simulink model "pitchShifter"  (R2020a)
settings: Solver=FixedStepAuto  StartTime=0.0  StopTime=386.015  FixedStep=1/4000  RelTol=1e-3  EnableMultiTasking=on
settings Model: Creator=Ivan Vican  LastModifiedBy=Korisnik
settings DataIOCC: LimitDataPoints=on  SaveFormat=Array  ReturnWorkspaceOutputs=off
settings OptimizationCC: ZeroExternalMemoryAtStartup=off  ZeroInternalMemoryAtStartup=off  LifeSpan=inf
settings DebuggingCC: SFUnexpectedBacktrackingDiag=warning  SFNoUnconditionalDefaultTransitionDiag=warning  ArithmeticOperatorsInVariantConditions=warning
settings HardwareCC: ProdBitPerPointer=32  ProdBitPerSizeT=32  ProdBitPerPtrDiffT=32  ProdLargestAtomicFloat=None  ProdIntDivRoundTo=Undefined  ProdEndianess=Unspecified  ProdWordSize=32  ProdHWDeviceType=32-bit Generic
settings ModelReferenceCC: PropagateSignalLabelsOutOfModel=off
settings SFSimCC: SimUseLocalCustomCode=off  CustomCodeUndefinedFunction=UseInterfaceOnly
settings RTWCC: RTWUseLocalCustomCode=off  TargetLang=C++
settings CodeAppCC: StateflowObjectComments=on
settings GRTTargetCC: TargetLangStandard=C89/C90 (ANSI)  MatFileLogging=off  MultiInstanceERTCode=on  CodeInterfacePackaging=C++ class
settings ConfigComp: CovMetricSettings=dw  CovHtmlReporting=on  CovSaveCumulativeToWorkspaceVar=on  CovSaveSingleToWorkspaceVar=on  CovExternalEMLEnable=off

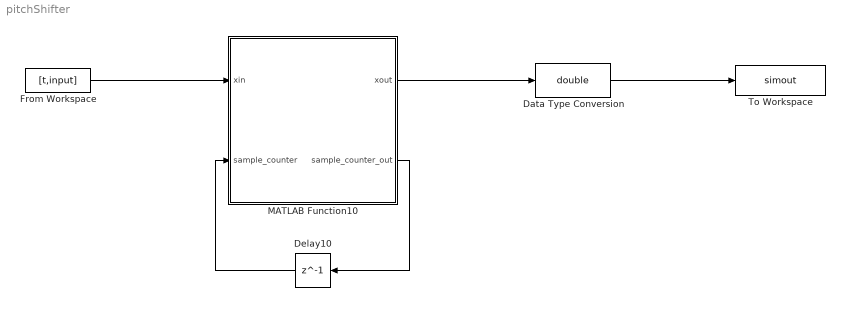
== system pitchShifter ==
  Data Type Conversion : DataTypeConversion  OutDataTypeStr=double
  Delay10 : Delay  DelayLength=1  InitialCondition=1
  From Workspace : FromWorkspace  VariableName=[t,input]  SampleTime=1/4000
  MATLAB Function10 : MATLAB Function  TreatAsAtomicUnit=on
  To Workspace : ToWorkspace  VariableName=simout  SampleTime=-1
      settings: Save2DSignal=2-D array (concatenate along first dimension)
  wires:
  Delay10/1 -> MATLAB Function10/2(sample_counter)
  MATLAB Function10/2(sample_counter_out) -> Delay10/1
  Data Type Conversion/1 -> To Workspace/1
  MATLAB Function10/1(xout) -> Data Type Conversion/1
  From Workspace/1 -> MATLAB Function10/1(xin)

== matlab function pitchShifter/MATLAB Function10 ==
  data: xin input; xout output; sample_counter input; sample_counter_out output
function [xout,sample_counter_out] = pitch24(xin,sample_counter)

persistent frame;
persistent frame_buff;
persistent frame_cnt;
persistent outputVector;
persistent pitchPrev;
persistent phaseCumulative;
persistent previousPhase;
persistent all;

% Window size
winSize = 128*2;
% Space between windows
hop = 8*2;
% Pitch scaling factor
alpha = 2^(24/12);
% Intermediate constants
hopOut = round(alpha*hop);

if isempty(frame)    
     frame = zeros([1,hop]);
     frame_buff = zeros([1,winSize]);
     frame_cnt = 0;
     outputVector = zeros([1,winSize]);
     pitchPrev = zeros([winSize/hop,winSize]);
     phaseCumulative = zeros(1,winSize);
     previousPhase = zeros(1,winSize);
     all = zeros([1,hop]);
end

frame(sample_counter) = xin;
xout = all(sample_counter);

% Intermediate constants
hopOut = round(alpha*hop);

% Hanning window for overlap-add
wn = hann(winSize*2+1);
wn = wn(2:2:end);

if sample_counter == hop
%% Initialization

% Create a frame matrix for the current input

% for i=1:winSize/hop-1
% pitchPrev(i,:) = pitchPrev(i+1,:);
% end

frame_cnt = frame_cnt + 1;

frame_buff = [frame_buff(hop+1:winSize) frame];
currentFrame = frame_buff;
    
%% Analysis
    
    % Window the frame
    currentFrameWindowed = currentFrame .* wn' / sqrt(((winSize/hop)/2));
    
    % Get the FFT
    currentFrameWindowedFFT = fft(currentFrameWindowed);
    
    % Get the magnitude
    magFrame = abs(currentFrameWindowedFFT);
    
    % Get the angle
    phaseFrame = angle(currentFrameWindowedFFT);
    
%% Processing    

    % Get the phase difference
    deltaPhi = phaseFrame - previousPhase;
    previousPhase = phaseFrame;
    
    % Remove the expected phase difference
    deltaPhiPrime = deltaPhi - hop * 2*pi*(0:(winSize-1))/winSize;
    
    % Map to -pi/pi range
    deltaPhiPrimeMod = mod(deltaPhiPrime+pi, 2*pi) - pi;
     
    % Get the true frequency
    trueFreq = 2*pi*(0:(winSize-1))/winSize + deltaPhiPrimeMod/hop;

    % Get the final phase
    phaseCumulative = phaseCumulative + hopOut * trueFreq;    
   
%% Synthesis    
    
    % Get the magnitude
    outputMag = magFrame;
    
    % Produce output frame
    outputFrame = real(ifft(outputMag .* exp(j*phaseCumulative)));
     
    % Save frame that has been processed
    outputy = outputFrame .* wn' / sqrt(((winSize/hopOut)/2));
       
  outputVector = outputy;
end

if (sample_counter == hop)
    sample_counter = 0;
    
    pitchPrev(mod(frame_cnt,winSize/hop)+1,:) = outputVector;
    
    outputStretched = zeros([1,hopOut]);
    
    for i=1:winSize/hopOut
    outputStretched = outputStretched + pitchPrev(mod(winSize/hop-i+1+frame_cnt,winSize/hop)+1,(i-1)*hopOut+1:i*hopOut);
    end
    
    all = interp1((0:(length(outputStretched)-1)),outputStretched,(0:alpha:(length(outputStretched)-1)),'linear');
 
end
sample_counter_out = sample_counter + 1;
    
end
